simulink model "Model_Control_system_SS"  (R2019a)
settings: Solver=FixedStepAuto  StartTime=0.0  StopTime=20  FixedStep=0.01  RelTol=1e-3
values from neighbouring files (symbols this model uses):
  K1 = acker(A1,B1,P1)    [Controller_system_SS.m]    (also in SS_controller_design.m)
  L1 = place(A1',C1',OP1)'    [Controller_system_SS.m]    (also in SS_controller_design.m)
undefined symbols (not defined in the file or in its folder): A1, B1, C1
settings Model: Creator=Tyson  LastModifiedBy=Tyson

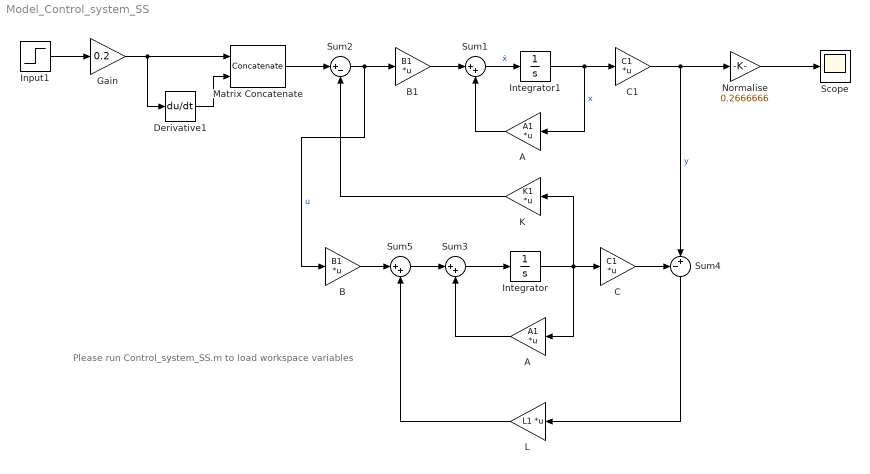
== system Model_Control_system_SS ==
  note: Please run Control_system_SS.m to load workspace variables
  "  A" : Gain  Gain=A1  Multiplication=Matrix(K*u)
  A : Gain  Gain=A1  Multiplication=Matrix(K*u)
  B : Gain  Gain=B1  Multiplication=Matrix(K*u)
  B1 : Gain  Gain=B1  Multiplication=Matrix(K*u)
  C : Gain  Gain=C1  Multiplication=Matrix(K*u)
  C1 : Gain  Gain=C1  Multiplication=Matrix(K*u)
  Derivative1 : Derivative
  "Gain " : Gain  Gain=0.2
  Input1 : Step  After=5  SampleTime=0
  Integrator : Integrator
  Integrator1 : Integrator
  K : Gain  Gain=K1  Multiplication=Matrix(K*u)
  L : Gain  Gain=L1  Multiplication=Matrix(K*u)
  Matrix Concatenate : Concatenate  Mode=Multidimensional array  ConcatenateDimension=2
  Normalise : Gain  Gain=0.2666666
  Scope : Scope
  Sum1 : Sum  Inputs=|++
  Sum2 : Sum  Inputs=|+-
  Sum3 : Sum  Inputs=|++
  Sum4 : Sum  Inputs=-+|
  Sum5 : Sum  Inputs=|++
  wires:
  Input1/1 -> "Gain "/1
  Derivative1/1 -> Matrix Concatenate/2
  C1/1 -> Normalise/1, Sum4/2  "y"
  Matrix Concatenate/1 -> Sum2/1
  Sum3/1 -> Integrator/1
  Integrator/1 -> C/1, "  A"/1, K/1
  K/1 -> Sum2/2
  Sum4/1 -> L/1
  "  A"/1 -> Sum3/2
  Sum5/1 -> Sum3/1
  L/1 -> Sum5/2
  C/1 -> Sum4/1
  B/1 -> Sum5/1
  "Gain "/1 -> Matrix Concatenate/1, Derivative1/1
  Normalise/1 -> Scope/1
  Sum2/1 -> B1/1, B/1  "u"
  A/1 -> Sum1/2
  Sum1/1 -> Integrator1/1  "ẋ"
  B1/1 -> Sum1/1
  Integrator1/1 -> C1/1, A/1  "x"
